simulink model "PID"  (R2021a)
settings: Solver=VariableStepAuto  StartTime=0  StopTime=10  RelTol=1e-3
values from neighbouring files (symbols this model uses):
  c1 = 1    [parameter.m]    (also in parameters.mat)
  c2 = 2    [parameter.m]    (also in parameters.mat)
  c3 = 3    [parameter.m]    (also in parameters.mat)
  g = 9.81    [parameter.m]    (also in parameters.mat)
  Ix = 1    [parameter.m]    (also in parameters.mat)
  Iy = 1    [parameter.m]    (also in parameters.mat)
  Iz = 1    [parameter.m]    (also in parameters.mat)
  k1 = 1    [parameter.m]    (also in parameters.mat)
  k2 = 2    [parameter.m]    (also in parameters.mat)
  k3 = 3    [parameter.m]    (also in parameters.mat)
  L = 1    [parameter.m]    (also in parameters.mat)
  m = 10    [parameter.m]    (also in parameters.mat)
libraries: pid_lib x1
settings Model: Creator=zlioo  LastModifiedBy=zlioo
settings DataIOCC: SaveFormat=StructureWithTime
settings OptimizationCC: BlockReduction=off  BufferReuse=off
settings DebuggingCC: AlgebraicLoopMsg=none  UnconnectedInputMsg=none  UnconnectedOutputMsg=none  UnconnectedLineMsg=none

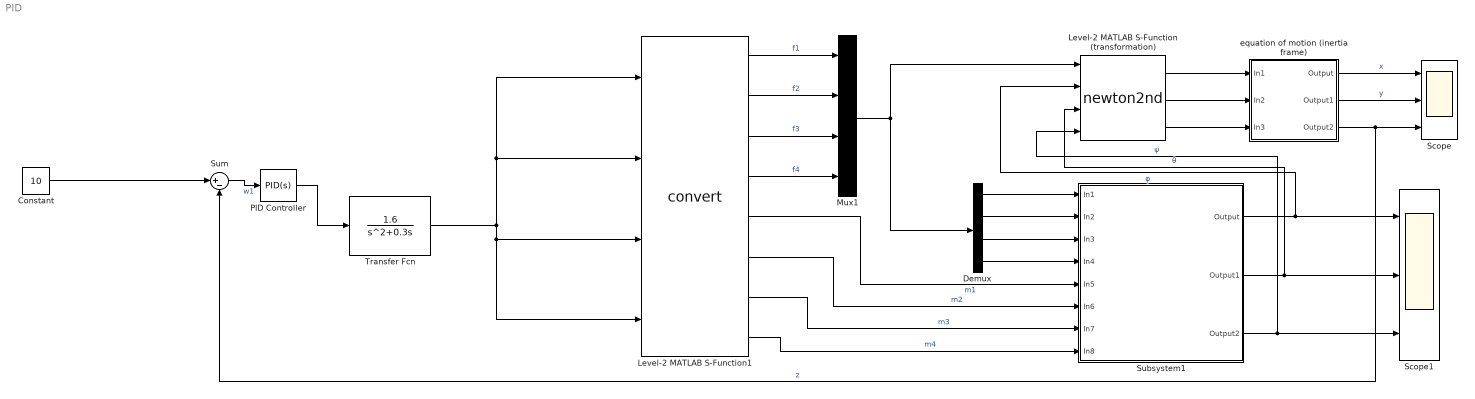
== system PID ==
  Constant : Constant  Value=10
  Demux : Demux
  Level-2 MATLAB S-Function (transformation) : M-S-Function  FunctionName=newton2nd
  Level-2 MATLAB S-Function1 : M-S-Function  FunctionName=convert
  Mux1 : Mux
  PID Controller : pid_lib/PID Controller  Controller=PID  Form=Parallel  TimeDomain=Continuous-time  UseExternalTs=off  SampleTime=-1  IntegratorMethod=Forward Euler  FilterMethod=Forward Euler  ControllerParametersSource=internal  P=1  I=1  D=0  UseFilter=on  N=100  TunerSelectOption=Transfer Function Based (PID Tuner App)  InitialConditionSource=internal  InitialConditionForIntegrator=0  InitialConditionForFilter=0  DifferentiatorICPrevScaledInput=0  ExternalReset=none  TrackingMode=off  Kt=1  LimitOutput=off  SatLimitsSource=internal  UpperSaturationLimit=inf  LowerSaturationLimit=-inf  LinearizeAsGain=on  AntiWindupMode=none  Kb=1  POutMin=[]  POutMax=[]  IOutMin=[]  IOutMax=[]  DOutMin=[]  DOutMax=[]  NOutMin=[]  NOutMax=[]  SumOutMin=[]  SumOutMax=[]  SaturationOutMin=[]  SaturationOutMax=[]  PParamMin=[]  PParamMax=[]  IParamMin=[]  IParamMax=[]  DParamMin=[]  DParamMax=[]  NParamMin=[]  NParamMax=[]  KbParamMin=[]  KbParamMax=[]  KtParamMin=[]  KtParamMax=[]  KbOutMin=[]  KbOutMax=[]  KtOutMin=[]  KtOutMax=[]  IntegratorOutMin=[]  IntegratorOutMax=[]  FilterOutMin=[]  FilterOutMax=[]  SumI1OutMin=[]  SumI1OutMax=[]  SumI2OutMin=[]  SumI2OutMax=[]  SumI3OutMin=[]  SumI3OutMax=[]  SumI4OutMin=[]  SumI4OutMax=[]  SumDOutMin=[]  SumDOutMax=[]  DifferentiatorOutMin=[]  DifferentiatorOutMax=[]  FilterDiffOutCoefMin=[]  FilterDiffOutCoefMax=[]  ReciprocalOutMin=[]  ReciprocalOutMax=[]  SumDenOutMin=[]  SumDenOutMax=[]  SumNumOutMin=[]  SumNumOutMax=[]  DivideOutMin=[]  DivideOutMax=[]  UdiffTsProdOutMin=[]  UdiffTsProdOutMax=[]  NTsProdOutMin=[]  NTsProdOutMax=[]  UintegralTsProdOutMin=[]  UintegralTsProdOutMax=[]  UngainTsProdOutMin=[]  UngainTsProdOutMax=[]  IntegratorContinuousStateAttributes=''  IntegratorStateMustResolveToSignalObject=off  IntegratorRTWStateStorageClass=Auto  FilterContinuousStateAttributes=''  FilterStateMustResolveToSignalObject=off  FilterRTWStateStorageClass=Auto  ParallelPVariant=InternalParameters  IdealPVariant=Disabled  IVariant=InternalParameters  DVariant=InternalParameters  IntegratorVariant=Continuous  SatVariant=Disabled  AWVariant=Passthrough  PCopyVariant=Disabled  TRVariant=Disabled  FdbkBlocksVariant=Forward  IdealPFdbkVariant=Disabled  SatFdbkVariant=Disabled  DerivativeFilterVariant=ContFilter  NVariant=InternalParameters  NCopyVariant=Disabled  FilterICVariant=InternalICsFilter  IntegratorICVariant=InternalICs  ExternalResetVariant=Disabled  TRSumVariant=Passthrough  SumFdbkVariant=Disabled  SumVariant=Sum_PID  TsampFilterVariant=InternalTs  TsampNgainVariant=Passthrough  TsampIntegralVariant=Passthrough  ExternalSaturationOutDataTypeStr=Inherit: Same as second input
  Scope : Scope  NumInputPorts=3
  Scope1 : Scope  NumInputPorts=3
  Subsystem1 : Subsystem
  Sum : Sum  Inputs=|+-
  Transfer Fcn : TransferFcn  Numerator=[1.6]  Denominator=[1 0.3 0]
  equation of motion (inertia frame) : Subsystem
  wires:
  Subsystem1/1(Output) -> Level-2 MATLAB S-Function (transformation)/2, Scope1/1  "φ"
  Level-2 MATLAB S-Function1/7 -> Subsystem1/7(In7)  "m3"
  equation of motion (inertia frame)/2(Output1) -> Scope/2  "y"
  Subsystem1/3(Output2) -> Level-2 MATLAB S-Function (transformation)/4, Scope1/3  "ψ"
  Level-2 MATLAB S-Function1/3 -> Mux1/3  "f3"
  Demux/2 -> Subsystem1/2(In2)
  Demux/1 -> Subsystem1/1(In1)
  Mux1/1 -> Demux/1, Level-2 MATLAB S-Function (transformation)/1
  equation of motion (inertia frame)/1(Output) -> Scope/1  "x"
  Level-2 MATLAB S-Function1/8 -> Subsystem1/8(In8)  "m4"
  Level-2 MATLAB S-Function1/6 -> Subsystem1/6(In6)  "m2"
  Level-2 MATLAB S-Function1/4 -> Mux1/4  "f4"
  Level-2 MATLAB S-Function (transformation)/3 -> equation of motion (inertia frame)/3(In3)
  Demux/4 -> Subsystem1/4(In4)
  equation of motion (inertia frame)/3(Output2) -> Scope/3, Sum/2  "z"
  Level-2 MATLAB S-Function1/1 -> Mux1/1  "f1"
  Level-2 MATLAB S-Function (transformation)/1 -> equation of motion (inertia frame)/1(In1)
  Subsystem1/2(Output1) -> Level-2 MATLAB S-Function (transformation)/3, Scope1/2  "θ"
  Level-2 MATLAB S-Function (transformation)/2 -> equation of motion (inertia frame)/2(In2)
  Demux/3 -> Subsystem1/3(In3)
  Level-2 MATLAB S-Function1/2 -> Mux1/2  "f2"
  Level-2 MATLAB S-Function1/5 -> Subsystem1/5(In5)  "m1"
  Constant/1 -> Sum/1
  Transfer Fcn/1 -> Level-2 MATLAB S-Function1/2, Level-2 MATLAB S-Function1/1, Level-2 MATLAB S-Function1/4, Level-2 MATLAB S-Function1/3
  Sum/1 -> PID Controller/1  "w1"
  PID Controller/1 -> Transfer Fcn/1

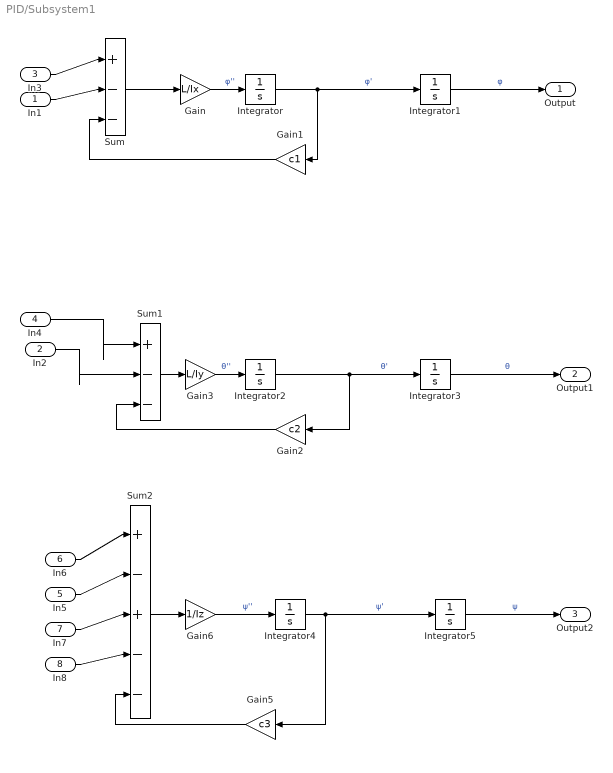
== system PID/Subsystem1 ==
  In1 : Inport
  In2 : Inport  Port=2
  In3 : Inport  Port=3
  In4 : Inport  Port=4
  In5 : Inport  Port=5
  In6 : Inport  Port=6
  In7 : Inport  Port=7
  In8 : Inport  Port=8
  Gain : Gain  Gain=L/Ix
  Gain1 : Gain  Gain=c1
  Gain2 : Gain  Gain=c2
  Gain3 : Gain  Gain=L/Iy
  Gain5 : Gain  Gain=c3
  Gain6 : Gain  Gain=1/Iz
  Integrator{,1..5} (6 alike) : Integrator
  Sum : Sum  Inputs=|+--
  Sum1 : Sum  Inputs=|+--
  Sum2 : Sum  Inputs=|+-+--
  Output : Outport
  Output1 : Outport  Port=2
  Output2 : Outport  Port=3
  wires:
  Integrator/1 -> Gain1/1, Integrator1/1  "φ'"
  Integrator2/1 -> Gain2/1, Integrator3/1  "θ'"
  Integrator4/1 -> Gain5/1, Integrator5/1  "ψ'"
  Integrator1/1 -> Output/1  "φ"
  Integrator3/1 -> Output1/1  "θ"
  Integrator5/1 -> Output2/1  "ψ"
  Gain6/1 -> Integrator4/1  "ψ''"
  In3/1 -> Sum/1
  In1/1 -> Sum/2
  Gain1/1 -> Sum/3
  Sum/1 -> Gain/1
  Gain/1 -> Integrator/1  "φ''"
  Gain2/1 -> Sum1/3
  In2/1 -> Sum1/2
  In4/1 -> Sum1/1
  Sum1/1 -> Gain3/1
  Gain3/1 -> Integrator2/1  "θ''"
  In6/1 -> Sum2/1
  In5/1 -> Sum2/2
  In7/1 -> Sum2/3
  In8/1 -> Sum2/4
  Gain5/1 -> Sum2/5
  Sum2/1 -> Gain6/1

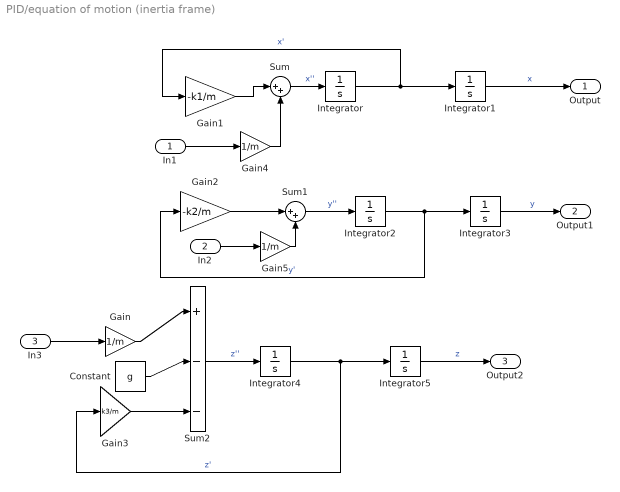
== system PID/equation of motion (inertia frame) ==
  In1 : Inport
  In2 : Inport  Port=2
  In3 : Inport  Port=3
  Constant : Constant  Value=g
  Gain : Gain  Gain=1/m
  Gain1 : Gain  Gain=-k1/m
  Gain2 : Gain  Gain=-k2/m
  Gain3 : Gain  Gain=k3/m
  Gain4 : Gain  Gain=1/m
  Gain5 : Gain  Gain=1/m
  Integrator{,1..5} (6 alike) : Integrator
  Sum : Sum  Inputs=|++
  Sum1 : Sum  Inputs=|++
  Sum2 : Sum  Inputs=|+--
  Output : Outport
  Output1 : Outport  Port=2
  Output2 : Outport  Port=3
  wires:
  Integrator/1 -> Gain1/1, Integrator1/1  "x'"
  Integrator2/1 -> Gain2/1, Integrator3/1  "y'"
  Integrator4/1 -> Integrator5/1, Gain3/1  "z'"
  Sum/1 -> Integrator/1  "x''"
  Gain1/1 -> Sum/1
  Gain2/1 -> Sum1/1
  Sum1/1 -> Integrator2/1  "y''"
  Integrator1/1 -> Output/1  "x"
  Integrator3/1 -> Output1/1  "y"
  Integrator5/1 -> Output2/1  "z"
  In3/1 -> Gain/1
  Gain/1 -> Sum2/1
  Constant/1 -> Sum2/2
  Gain3/1 -> Sum2/3
  Sum2/1 -> Integrator4/1  "z''"
  In1/1 -> Gain4/1
  Gain4/1 -> Sum/2
  In2/1 -> Gain5/1
  Gain5/1 -> Sum1/2
